simulink model "Sense"  (R2020a)
settings: Solver=FixedStepAuto  StartTime=0.0  StopTime=10.0  FixedStep=1e-3  RelTol=1e-3  EnableMultiTasking=on
undefined symbols (not defined in the file): D0, D1, D13, D3, D6, PTA1, PTC16, PTC17, PTC2, PTD1
libraries: frdmk64flib x7, simulink x2
settings Model: ExtModeTrigDuration=5  Creator=WinnieTrandinh  LastModifiedBy=Liam
settings OptimizationCC: EnhancedBackFolding=on  PassReuseOutputArgsAs=Individual arguments  ZeroExternalMemoryAtStartup=off  ZeroInternalMemoryAtStartup=off  MaxStackSize=64  OptimizeBlockOrder=speed  DifferentSizesBufferReuse=on  OptimizationCustomize=off  EfficientTunableParamExpr=on
settings DebuggingCC: ParameterTunabilityLossMsg=error
settings HardwareCC: ProdBitPerPointer=32  ProdBitPerSizeT=32  ProdBitPerPtrDiffT=32  ProdLargestAtomicInteger=Long  ProdLargestAtomicFloat=Double  ProdWordSize=32  ProdHWDeviceType=ARM Compatible->ARM Cortex
settings SFSimCC: MATLABDynamicMemAlloc=off
settings RTWCC: SystemTargetFile=ert.tlc  HardwareBoard=NXP FRDM-K64F  TemplateMakefile=ert_default_tmf  Toolchain=GNU Tools for ARM Embedded Processors
settings CodeAppCC: ForceParamTrailComments=on  IgnoreCustomStorageClasses=off  OperatorAnnotations=on  SimulinkDataObjDesc=on  SFDataObjDesc=on  InsertBlockDesc=on

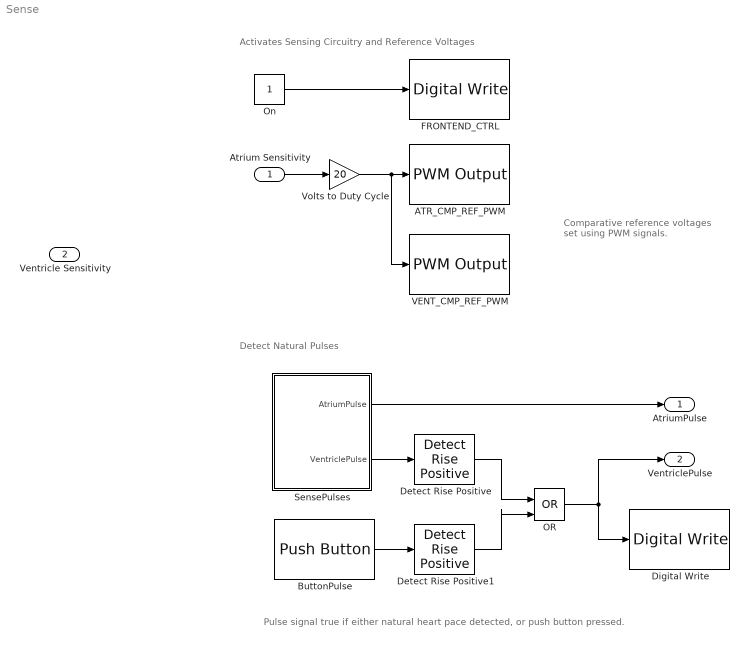
== system Sense ==
  note: Pulse signal true if either natural heart pace detected, or push button pressed.
  note: Comparative reference voltages
      | set using PWM signals.
  note: Detect Natural Pulses
  note: Activates Sensing Circuitry and Reference Voltages
  " Atrium Sensitivity" : Inport  Unit=volt
  Ventricle Sensitivity : Inport  Port=2
  ATR_CMP_REF_PWM : frdmk64flib/PWM Output  Whichpin=PTC2 (D6)  InitialFrequency=2000  InitialDutyCycle=20
  ButtonPulse : frdmk64flib/Push Button  Whichswitch=SW2  SampleTime1=-1
  Detect Rise Positive : simulink/Logic and Bit Operations/Detect Rise Positive  vinit=0  OutDataTypeStr=boolean
  Detect Rise Positive1 : simulink/Logic and Bit Operations/Detect Rise Positive  vinit=0  OutDataTypeStr=boolean
  Digital Write : frdmk64flib/Digital Write  Whichpin=RED_LED
  FRONTEND_CTRL : frdmk64flib/Digital Write  Whichpin=PTD1 (D13)
  OR : Logic  Operator=OR  IconShape=distinctive  AllPortsSameDT=off  OutDataTypeStr=boolean
  On : Constant
  SensePulses : Subsystem  Variant=on
  "VENT_CMP_REF_PWM " : frdmk64flib/PWM Output  Whichpin=PTA1 (D3)  InitialFrequency=2000  InitialDutyCycle=20
  Volts to Duty Cycle : Gain  Gain=20
  AtriumPulse : Outport
  VentriclePulse : Outport  Port=2
  wires:
  On/1 -> FRONTEND_CTRL/1
  SensePulses/2(VentriclePulse) -> Detect Rise Positive/1
  OR/1 -> VentriclePulse/1, Digital Write/1
  ButtonPulse/1 -> Detect Rise Positive1/1
  Detect Rise Positive/1 -> OR/1
  Detect Rise Positive1/1 -> OR/2
  Volts to Duty Cycle/1 -> "VENT_CMP_REF_PWM "/1, ATR_CMP_REF_PWM/1
  " Atrium Sensitivity"/1 -> Volts to Duty Cycle/1
  SensePulses/1(AtriumPulse) -> AtriumPulse/1

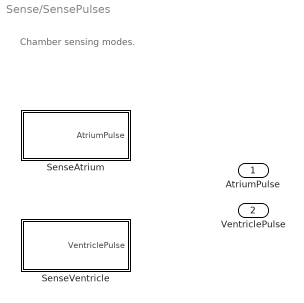
== system Sense/SensePulses ==
  note: Chamber sensing modes.
  SenseAtrium : Subsystem  VariantControl=ATR_SENSING
  SenseVentricle : Subsystem  VariantControl=VENT_SENSING
  AtriumPulse : Outport
  VentriclePulse : Outport  Port=2

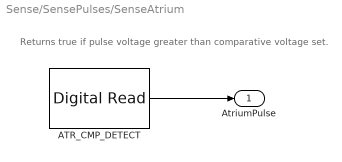
== system Sense/SensePulses/SenseAtrium ==
  note: Returns true if pulse voltage greater than comparative voltage set.
  ATR_CMP_DETECT : frdmk64flib/Digital Read  Whichpin=PTC16 (D0)  SampleTime=-1
  AtriumPulse : Outport
  wires:
  ATR_CMP_DETECT/1 -> AtriumPulse/1

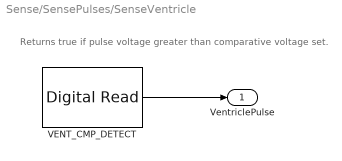
== system Sense/SensePulses/SenseVentricle ==
  note: Returns true if pulse voltage greater than comparative voltage set.
  VENT_CMP_DETECT : frdmk64flib/Digital Read  Whichpin=PTC17 (D1)  SampleTime=-1
  VentriclePulse : Outport
  wires:
  VENT_CMP_DETECT/1 -> VentriclePulse/1
